simulink model "problem4_ex3"  (R2020a)
settings: Solver=VariableStepAuto  StartTime=0.0  StopTime=10.0  RelTol=1e-3
settings Model: Creator=dinhm  LastModifiedBy=dinhm

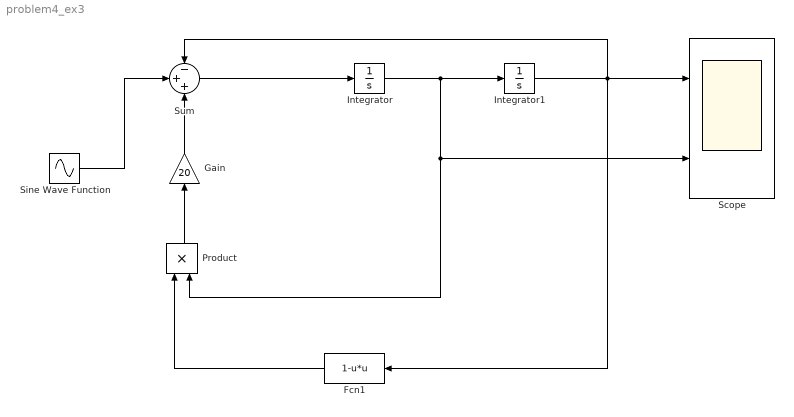
== system problem4_ex3 ==
  Fcn1 : Fcn  Expr=1-u*u
  Gain : Gain  Gain=20
  Integrator : Integrator
  Integrator1 : Integrator  InitialCondition=2
  Product : Product
  Scope : Scope  NumInputPorts=2
  Sine Wave Function : Sin  TimeSource=Use external signal  Amplitude=0.5  Phase=pi/2  SampleTime=0
  Sum : Sum  Inputs=-++
  wires:
  Sum/1 -> Integrator/1
  Integrator/1 -> Product/2, Scope/2, Integrator1/1
  Integrator1/1 -> Fcn1/1, Scope/1, Sum/1
  Product/1 -> Gain/1
  Fcn1/1 -> Product/1
  Gain/1 -> Sum/3
  Sine Wave Function/1 -> Sum/2
